simulink model "SmaSimulink"  (R2018a)
settings: Solver=FixedStepAuto  StartTime=0.0  StopTime=2  FixedStep=10e-6  RelTol=1e-6
values from neighbouring files (symbols this model uses):
  Af = 80 - ABS_ZERO_TEMP    (= 353.15)    [TempBris.m]    (also in TensileSMA.m = 353)
  As = 70 - ABS_ZERO_TEMP    (= 343.15)    [TempBris.m]    (also in TensileSMA.m = 343)
  Ca = 13.8 * 10^6    (= 13800000)    [TensileSMA.m]
  Cm = 8 * 10^6    (= 8000000)    [TensileSMA.m]
  cSf = 170 * 10^6    (= 170000000)    [TensileSMA.m]
  cSs = 100 * 10^6    (= 100000000)    [TensileSMA.m]
  Da = 6.7 * 10^4 * 10^6    (= 67000000000)    [TensileSMA.m]
  Dm = 2.63 * 10^4 * 10^6    (= 26300000000)    [TensileSMA.m]
  Mf = 40 - ABS_ZERO_TEMP    (= 313.15)    [TempBris.m]    (also in TensileSMA.m = 313)
  Ms = 50 - ABS_ZERO_TEMP    (= 323.15)    [TempBris.m]    (also in TensileSMA.m = 323)
  rEmax = 0.05    [TensileSMA.m]
undefined symbols (not defined in the file or in its folder): martDetwiningStrain, martDetwiningStress, sigma, simout, strain_mart, stress_mart, stressSweep, temp_mart_out
libraries: powerlib_meascontrol x1
(part 2 of 2)

== system SmaSimulink/Subsystem/Antagonistic /T < Mf2/T < Mf SigmaCritS < T < SigmaCritF ==
  Xi_s_in : Inport
  Sigma : Inport  Port=2
  Add1 : Sum  Inputs=+-
  Add3 : Sum
  Constant1 : Constant  Value=cSf
  Constant2 : Constant  Value=pi/(cSs-cSf)
  Cos : Trigonometry  Operator=cos
  Product2 : Product
  Product3 : Product
  "[(1+x)/2]" : Subsystem
  "[(1-x)/2]" : Subsystem
  Xi_t_out : Outport
  wires:
  Cos/1 -> Product2/2
  Product2/1 -> Add3/2
  Add1/1 -> Product3/2
  Sigma/1 -> Add1/1
  Add3/1 -> Xi_t_out/1
  Xi_s_in/1 -> "[(1+x)/2]"/1(In), "[(1-x)/2]"/1(In)
  Product3/1 -> Cos/1
  "[(1+x)/2]"/1(Out) -> Add3/1
  "[(1-x)/2]"/1(Out) -> Product2/1
  Constant2/1 -> Product3/1
  Constant1/1 -> Add1/2

== system SmaSimulink/Subsystem/Ms < T <  As SigmaCritF > Sigma > SigmaCritS/T > Ms Xi_s/[(1+x)//2] ==
  In : Inport
  Add1 : Sum
  Constant1 : Constant
  Constant3 : Constant  Value=2
  Divide1 : Product  Inputs=*/
  Out : Outport
  wires:
  Constant3/1 -> Divide1/2
  Divide1/1 -> Out/1
  Constant1/1 -> Add1/1
  In/1 -> Add1/2
  Add1/1 -> Divide1/1

== system SmaSimulink/Subsystem/Ms < T <  As SigmaCritF > Sigma > SigmaCritS/T > Ms Xi_s/[(1-x)//2] ==
  In : Inport
  Add1 : Sum  Inputs=+-
  Constant1 : Constant
  Constant3 : Constant  Value=2
  Divide1 : Product  Inputs=*/
  Out : Outport
  wires:
  Constant3/1 -> Divide1/2
  Divide1/1 -> Out/1
  Constant1/1 -> Add1/1
  In/1 -> Add1/2
  Add1/1 -> Divide1/1

== system SmaSimulink/Subsystem/Strain(Stress) Constitute/Subsystem1/Subsystem1 ==
  Xi : Inport
  Add : Sum
  Constant : Constant  Value=Dm-Da
  Constant1 : Constant  Value=Da
  Product : Product
  D : Outport
  wires:
  Xi/1 -> Product/2
  Product/1 -> Add/1
  Constant1/1 -> Add/2
  Constant/1 -> Product/1
  Add/1 -> D/1

== system SmaSimulink/Subsystem/Strain(Stress) Constitute/Subsystem2/Subsystem1 ==
  Xi : Inport
  Add : Sum
  Constant : Constant  Value=Dm-Da
  Constant1 : Constant  Value=Da
  Product : Product
  D : Outport
  wires:
  Xi/1 -> Product/2
  Product/1 -> Add/1
  Constant1/1 -> Add/2
  Constant/1 -> Product/1
  Add/1 -> D/1

== system SmaSimulink/Subsystem/Strain(Stress) Constitute1/Subsystem1/Subsystem1 ==
  Xi : Inport
  Add : Sum
  Constant : Constant  Value=Dm-Da
  Constant1 : Constant  Value=Da
  Product : Product
  D : Outport
  wires:
  Xi/1 -> Product/2
  Product/1 -> Add/1
  Constant1/1 -> Add/2
  Constant/1 -> Product/1
  Add/1 -> D/1

== system SmaSimulink/Subsystem/Strain(Stress) Constitute1/Subsystem2/Subsystem1 ==
  Xi : Inport
  Add : Sum
  Constant : Constant  Value=Dm-Da
  Constant1 : Constant  Value=Da
  Product : Product
  D : Outport
  wires:
  Xi/1 -> Product/2
  Product/1 -> Add/1
  Constant1/1 -> Add/2
  Constant/1 -> Product/1
  Add/1 -> D/1

== system SmaSimulink/Subsystem/Stress(Strain) Constitute/Subsystem1/Subsystem1 ==
  Xi : Inport
  Add : Sum
  Constant : Constant  Value=Dm-Da
  Constant1 : Constant  Value=Da
  Product : Product
  D : Outport
  wires:
  Xi/1 -> Product/2
  Product/1 -> Add/1
  Constant1/1 -> Add/2
  Constant/1 -> Product/1
  Add/1 -> D/1

== system SmaSimulink/Subsystem/Stress(Strain) Constitute/Subsystem2/Subsystem1 ==
  Xi : Inport
  Add : Sum
  Constant : Constant  Value=Dm-Da
  Constant1 : Constant  Value=Da
  Product : Product
  D : Outport
  wires:
  Xi/1 -> Product/2
  Product/1 -> Add/1
  Constant1/1 -> Add/2
  Constant/1 -> Product/1
  Add/1 -> D/1

== system SmaSimulink/Subsystem/Stress(Strain) Constitute1/Subsystem1/Subsystem1 ==
  Xi : Inport
  Add : Sum
  Constant : Constant  Value=Dm-Da
  Constant1 : Constant  Value=Da
  Product : Product
  D : Outport
  wires:
  Xi/1 -> Product/2
  Product/1 -> Add/1
  Constant1/1 -> Add/2
  Constant/1 -> Product/1
  Add/1 -> D/1

== system SmaSimulink/Subsystem/Stress(Strain) Constitute1/Subsystem2/Subsystem1 ==
  Xi : Inport
  Add : Sum
  Constant : Constant  Value=Dm-Da
  Constant1 : Constant  Value=Da
  Product : Product
  D : Outport
  wires:
  Xi/1 -> Product/2
  Product/1 -> Add/1
  Constant1/1 -> Add/2
  Constant/1 -> Product/1
  Add/1 -> D/1

== system SmaSimulink/Subsystem/Stress(Strain) Constitute2/Subsystem1/Subsystem1 ==
  Xi : Inport
  Add : Sum
  Constant : Constant  Value=Dm-Da
  Constant1 : Constant  Value=Da
  Product : Product
  D : Outport
  wires:
  Xi/1 -> Product/2
  Product/1 -> Add/1
  Constant1/1 -> Add/2
  Constant/1 -> Product/1
  Add/1 -> D/1

== system SmaSimulink/Subsystem/Stress(Strain) Constitute2/Subsystem2/Subsystem1 ==
  Xi : Inport
  Add : Sum
  Constant : Constant  Value=Dm-Da
  Constant1 : Constant  Value=Da
  Product : Product
  D : Outport
  wires:
  Xi/1 -> Product/2
  Product/1 -> Add/1
  Constant1/1 -> Add/2
  Constant/1 -> Product/1
  Add/1 -> D/1

== system SmaSimulink/Subsystem/Subsystem1/Af > T > As1/T > As Xi  ==
  Xi_in : Inport
  T : Inport  Port=2
  "Sigma " : Inport  Port=3
  Add1 : Sum  Inputs=+--
  Add2 : Sum
  Constant1 : Constant  Value=Ca
  Constant2 : Constant  Value=pi/(Af-As)
  Constant3 : Constant
  Constant4 : Constant  Value=As
  Constant5 : Constant  Value=2
  Cos : Trigonometry  Operator=cos
  Divide : Product  Inputs=*/
  Divide1 : Product  Inputs=*/
  Product1 : Product
  Product3 : Product
  Xi_out : Outport
  wires:
  Constant4/1 -> Add1/2
  Xi_in/1 -> Divide1/1
  T/1 -> Add1/1
  Add1/1 -> Product3/2
  Constant2/1 -> Product3/1
  Product3/1 -> Cos/1
  "Sigma "/1 -> Divide/1
  Constant1/1 -> Divide/2
  Divide/1 -> Add1/3
  Cos/1 -> Add2/1
  Constant3/1 -> Add2/2
  Constant5/1 -> Divide1/2
  Add2/1 -> Product1/2
  Divide1/1 -> Product1/1
  Product1/1 -> Xi_out/1

== system SmaSimulink/Subsystem/Subsystem1/Af > T > As1/T > As Xi_s ==
  "Xi_s_in " : Inport
  Xi_in : Inport  Port=2
  Xi_out : Inport  Port=3
  Add1 : Sum  Inputs=+-
  Add2 : Sum  Inputs=+-
  Divide : Product  Inputs=*/
  Product1 : Product
  Scope : Scope
  Xi_s_out : Outport
  wires:
  Xi_in/1 -> Add2/1, Divide/2
  "Xi_s_in "/1 -> Add1/1, Divide/1
  Add1/1 -> Xi_s_out/1
  Xi_out/1 -> Add2/2
  Divide/1 -> Product1/1
  Add2/1 -> Scope/1, Product1/2
  Product1/1 -> Add1/2

== system SmaSimulink/Subsystem/Subsystem1/Af > T > As1/T > As Xi_t ==
  "Xi_t_in " : Inport
  Xi_in : Inport  Port=2
  Xi_out : Inport  Port=3
  Add1 : Sum  Inputs=+-
  Add2 : Sum  Inputs=+-
  Divide : Product  Inputs=*/
  Product1 : Product
  Xi_t_out : Outport
  wires:
  Xi_in/1 -> Add2/1, Divide/2
  "Xi_t_in "/1 -> Add1/1, Divide/1
  Add1/1 -> Xi_t_out/1
  Xi_out/1 -> Add2/2
  Divide/1 -> Product1/1
  Add2/1 -> Product1/2
  Product1/1 -> Add1/2

== system SmaSimulink/Subsystem/Subsystem2/Af > T > As1/T > As Xi  ==
  Xi_in : Inport
  T : Inport  Port=2
  "Sigma " : Inport  Port=3
  Add1 : Sum  Inputs=+--
  Add2 : Sum
  Constant1 : Constant  Value=Ca
  Constant2 : Constant  Value=pi/(Af-As)
  Constant3 : Constant
  Constant4 : Constant  Value=As
  Constant5 : Constant  Value=2
  Cos : Trigonometry  Operator=cos
  Divide : Product  Inputs=*/
  Divide1 : Product  Inputs=*/
  Product1 : Product
  Product3 : Product
  Xi_out : Outport
  wires:
  Constant4/1 -> Add1/2
  Xi_in/1 -> Divide1/1
  T/1 -> Add1/1
  Add1/1 -> Product3/2
  Constant2/1 -> Product3/1
  Product3/1 -> Cos/1
  "Sigma "/1 -> Divide/1
  Constant1/1 -> Divide/2
  Divide/1 -> Add1/3
  Cos/1 -> Add2/1
  Constant3/1 -> Add2/2
  Constant5/1 -> Divide1/2
  Add2/1 -> Product1/2
  Divide1/1 -> Product1/1
  Product1/1 -> Xi_out/1

== system SmaSimulink/Subsystem/Subsystem2/Af > T > As1/T > As Xi_s ==
  "Xi_s_in " : Inport
  Xi_in : Inport  Port=2
  Xi_out : Inport  Port=3
  Add1 : Sum  Inputs=+-
  Add2 : Sum  Inputs=+-
  Divide : Product  Inputs=*/
  Product1 : Product
  Xi_s_out : Outport
  wires:
  Xi_in/1 -> Add2/1, Divide/2
  "Xi_s_in "/1 -> Add1/1, Divide/1
  Add1/1 -> Xi_s_out/1
  Xi_out/1 -> Add2/2
  Divide/1 -> Product1/1
  Add2/1 -> Product1/2
  Product1/1 -> Add1/2

== system SmaSimulink/Subsystem/Subsystem2/Af > T > As1/T > As Xi_t ==
  "Xi_t_in " : Inport
  Xi_in : Inport  Port=2
  Xi_out : Inport  Port=3
  Add1 : Sum  Inputs=+-
  Add2 : Sum  Inputs=+-
  Divide : Product  Inputs=*/
  Product1 : Product
  Xi_t_out : Outport
  wires:
  Xi_in/1 -> Add2/1, Divide/2
  "Xi_t_in "/1 -> Add1/1, Divide/1
  Add1/1 -> Xi_t_out/1
  Xi_out/1 -> Add2/2
  Divide/1 -> Product1/1
  Add2/1 -> Product1/2
  Product1/1 -> Add1/2

== system SmaSimulink/Subsystem/T < Mf/T < Mf SigmaCritS < T < SigmaCritF/[(1+x)//2] ==
  In : Inport
  Add1 : Sum
  Constant1 : Constant
  Constant3 : Constant  Value=2
  Divide1 : Product  Inputs=*/
  Out : Outport
  wires:
  Constant3/1 -> Divide1/2
  Divide1/1 -> Out/1
  Constant1/1 -> Add1/1
  In/1 -> Add1/2
  Add1/1 -> Divide1/1

== system SmaSimulink/Subsystem/T < Mf/T < Mf SigmaCritS < T < SigmaCritF/[(1-x)//2] ==
  In : Inport
  Add1 : Sum  Inputs=+-
  Constant1 : Constant
  Constant3 : Constant  Value=2
  Divide1 : Product  Inputs=*/
  Out : Outport
  wires:
  Constant3/1 -> Divide1/2
  Divide1/1 -> Out/1
  Constant1/1 -> Add1/1
  In/1 -> Add1/2
  Add1/1 -> Divide1/1

== system SmaSimulink/Subsystem/T < Mf1/T < Mf SigmaCritS < T < SigmaCritF/[(1+x)//2] ==
  In : Inport
  Add1 : Sum
  Constant1 : Constant
  Constant3 : Constant  Value=2
  Divide1 : Product  Inputs=*/
  Out : Outport
  wires:
  Constant3/1 -> Divide1/2
  Divide1/1 -> Out/1
  Constant1/1 -> Add1/1
  In/1 -> Add1/2
  Add1/1 -> Divide1/1

== system SmaSimulink/Subsystem/T < Mf1/T < Mf SigmaCritS < T < SigmaCritF/[(1-x)//2] ==
  In : Inport
  Add1 : Sum  Inputs=+-
  Constant1 : Constant
  Constant3 : Constant  Value=2
  Divide1 : Product  Inputs=*/
  Out : Outport
  wires:
  Constant3/1 -> Divide1/2
  Divide1/1 -> Out/1
  Constant1/1 -> Add1/1
  In/1 -> Add1/2
  Add1/1 -> Divide1/1

== system SmaSimulink/Subsystem/T < Mf2/T < Mf SigmaCritS < T < SigmaCritF/[(1+x)//2] ==
  In : Inport
  Add1 : Sum
  Constant1 : Constant
  Constant3 : Constant  Value=2
  Divide1 : Product  Inputs=*/
  Out : Outport
  wires:
  Constant3/1 -> Divide1/2
  Divide1/1 -> Out/1
  Constant1/1 -> Add1/1
  In/1 -> Add1/2
  Add1/1 -> Divide1/1

== system SmaSimulink/Subsystem/T < Mf2/T < Mf SigmaCritS < T < SigmaCritF/[(1-x)//2] ==
  In : Inport
  Add1 : Sum  Inputs=+-
  Constant1 : Constant
  Constant3 : Constant  Value=2
  Divide1 : Product  Inputs=*/
  Out : Outport
  wires:
  Constant3/1 -> Divide1/2
  Divide1/1 -> Out/1
  Constant1/1 -> Add1/1
  In/1 -> Add1/2
  Add1/1 -> Divide1/1

== system SmaSimulink/Subsystem/T > As/Af > T > As1/T > As Xi  ==
  Xi_in : Inport
  T : Inport  Port=2
  "Sigma " : Inport  Port=3
  Add1 : Sum  Inputs=+--
  Add2 : Sum
  Constant1 : Constant  Value=Ca
  Constant2 : Constant  Value=pi/(Af-As)
  Constant3 : Constant
  Constant4 : Constant  Value=As
  Constant5 : Constant  Value=2
  Cos : Trigonometry  Operator=cos
  Divide : Product  Inputs=*/
  Divide1 : Product  Inputs=*/
  Product1 : Product
  Product3 : Product
  Xi_out : Outport
  wires:
  Constant4/1 -> Add1/2
  Xi_in/1 -> Divide1/1
  T/1 -> Add1/1
  Add1/1 -> Product3/2
  Constant2/1 -> Product3/1
  Product3/1 -> Cos/1
  "Sigma "/1 -> Divide/1
  Constant1/1 -> Divide/2
  Divide/1 -> Add1/3
  Cos/1 -> Add2/1
  Constant3/1 -> Add2/2
  Constant5/1 -> Divide1/2
  Add2/1 -> Product1/2
  Divide1/1 -> Product1/1
  Product1/1 -> Xi_out/1

== system SmaSimulink/Subsystem/T > As/Af > T > As1/T > As Xi_s ==
  "Xi_s_in " : Inport
  Xi_in : Inport  Port=2
  Xi_out : Inport  Port=3
  Add1 : Sum  Inputs=+-
  Add2 : Sum  Inputs=+-
  Divide : Product  Inputs=*/
  Product1 : Product
  Xi_s_out : Outport
  wires:
  Xi_in/1 -> Add2/1, Divide/2
  "Xi_s_in "/1 -> Add1/1, Divide/1
  Add1/1 -> Xi_s_out/1
  Xi_out/1 -> Add2/2
  Divide/1 -> Product1/1
  Add2/1 -> Product1/2
  Product1/1 -> Add1/2

== system SmaSimulink/Subsystem/T > As/Af > T > As1/T > As Xi_t ==
  "Xi_t_in " : Inport
  Xi_in : Inport  Port=2
  Xi_out : Inport  Port=3
  Add1 : Sum  Inputs=+-
  Add2 : Sum  Inputs=+-
  Divide : Product  Inputs=*/
  Product1 : Product
  Xi_t_out : Outport
  wires:
  Xi_in/1 -> Add2/1, Divide/2
  "Xi_t_in "/1 -> Add1/1, Divide/1
  Add1/1 -> Xi_t_out/1
  Xi_out/1 -> Add2/2
  Divide/1 -> Product1/1
  Add2/1 -> Product1/2
  Product1/1 -> Add1/2

== system SmaSimulink/Subsystem/Antagonistic /Strain(Stress) Constitute1/Subsystem1/Subsystem1 ==
  Xi : Inport
  Add : Sum
  Constant : Constant  Value=Dm-Da
  Constant1 : Constant  Value=Da
  Product : Product
  D : Outport
  wires:
  Xi/1 -> Product/2
  Product/1 -> Add/1
  Constant1/1 -> Add/2
  Constant/1 -> Product/1
  Add/1 -> D/1

== system SmaSimulink/Subsystem/Antagonistic /Strain(Stress) Constitute1/Subsystem2/Subsystem1 ==
  Xi : Inport
  Add : Sum
  Constant : Constant  Value=Dm-Da
  Constant1 : Constant  Value=Da
  Product : Product
  D : Outport
  wires:
  Xi/1 -> Product/2
  Product/1 -> Add/1
  Constant1/1 -> Add/2
  Constant/1 -> Product/1
  Add/1 -> D/1

== system SmaSimulink/Subsystem/Antagonistic /Stress(Strain) Constitute1/Subsystem1/Subsystem1 ==
  Xi : Inport
  Add : Sum
  Constant : Constant  Value=Dm-Da
  Constant1 : Constant  Value=Da
  Product : Product
  D : Outport
  wires:
  Xi/1 -> Product/2
  Product/1 -> Add/1
  Constant1/1 -> Add/2
  Constant/1 -> Product/1
  Add/1 -> D/1

== system SmaSimulink/Subsystem/Antagonistic /Stress(Strain) Constitute1/Subsystem2/Subsystem1 ==
  Xi : Inport
  Add : Sum
  Constant : Constant  Value=Dm-Da
  Constant1 : Constant  Value=Da
  Product : Product
  D : Outport
  wires:
  Xi/1 -> Product/2
  Product/1 -> Add/1
  Constant1/1 -> Add/2
  Constant/1 -> Product/1
  Add/1 -> D/1

== system SmaSimulink/Subsystem/Antagonistic /Subsystem3/Af > T > As1/T > As Xi  ==
  Xi_in : Inport
  T : Inport  Port=2
  "Sigma " : Inport  Port=3
  Add1 : Sum  Inputs=+--
  Add2 : Sum
  Constant1 : Constant  Value=Ca
  Constant2 : Constant  Value=pi/(Af-As)
  Constant3 : Constant
  Constant4 : Constant  Value=As
  Constant5 : Constant  Value=2
  Cos : Trigonometry  Operator=cos
  Divide : Product  Inputs=*/
  Divide1 : Product  Inputs=*/
  Product1 : Product
  Product3 : Product
  Xi_out : Outport
  wires:
  Constant4/1 -> Add1/2
  Xi_in/1 -> Divide1/1
  T/1 -> Add1/1
  Add1/1 -> Product3/2
  Constant2/1 -> Product3/1
  Product3/1 -> Cos/1
  "Sigma "/1 -> Divide/1
  Constant1/1 -> Divide/2
  Divide/1 -> Add1/3
  Cos/1 -> Add2/1
  Constant3/1 -> Add2/2
  Constant5/1 -> Divide1/2
  Add2/1 -> Product1/2
  Divide1/1 -> Product1/1
  Product1/1 -> Xi_out/1

== system SmaSimulink/Subsystem/Antagonistic /Subsystem3/Af > T > As1/T > As Xi_s ==
  "Xi_s_in " : Inport
  Xi_in : Inport  Port=2
  Xi_out : Inport  Port=3
  Add1 : Sum  Inputs=+-
  Add2 : Sum  Inputs=+-
  Divide : Product  Inputs=*/
  Product1 : Product
  Xi_s_out : Outport
  wires:
  Xi_in/1 -> Add2/1, Divide/2
  "Xi_s_in "/1 -> Add1/1, Divide/1
  Add1/1 -> Xi_s_out/1
  Xi_out/1 -> Add2/2
  Divide/1 -> Product1/1
  Add2/1 -> Product1/2
  Product1/1 -> Add1/2

== system SmaSimulink/Subsystem/Antagonistic /Subsystem3/Af > T > As1/T > As Xi_t ==
  "Xi_t_in " : Inport
  Xi_in : Inport  Port=2
  Xi_out : Inport  Port=3
  Add1 : Sum  Inputs=+-
  Add2 : Sum  Inputs=+-
  Divide : Product  Inputs=*/
  Product1 : Product
  Xi_t_out : Outport
  wires:
  Xi_in/1 -> Add2/1, Divide/2
  "Xi_t_in "/1 -> Add1/1, Divide/1
  Add1/1 -> Xi_t_out/1
  Xi_out/1 -> Add2/2
  Divide/1 -> Product1/1
  Add2/1 -> Product1/2
  Product1/1 -> Add1/2

== system SmaSimulink/Subsystem/Antagonistic /T < Mf2/T < Mf SigmaCritS < T < SigmaCritF/[(1+x)//2] ==
  In : Inport
  Add1 : Sum
  Constant1 : Constant
  Constant3 : Constant  Value=2
  Divide1 : Product  Inputs=*/
  Out : Outport
  wires:
  Constant3/1 -> Divide1/2
  Divide1/1 -> Out/1
  Constant1/1 -> Add1/1
  In/1 -> Add1/2
  Add1/1 -> Divide1/1

== system SmaSimulink/Subsystem/Antagonistic /T < Mf2/T < Mf SigmaCritS < T < SigmaCritF/[(1-x)//2] ==
  In : Inport
  Add1 : Sum  Inputs=+-
  Constant1 : Constant
  Constant3 : Constant  Value=2
  Divide1 : Product  Inputs=*/
  Out : Outport
  wires:
  Constant3/1 -> Divide1/2
  Divide1/1 -> Out/1
  Constant1/1 -> Add1/1
  In/1 -> Add1/2
  Add1/1 -> Divide1/1
